simulink library "lineAngleSensorObserver"  (R2022a)
settings: Solver=VariableStepAuto  StartTime=0.0  StopTime=10.0  RelTol=1e-3
undefined symbols (not defined in the file): accelBias, bridlePosVec, env, eulerBias, fluidDensity, gravity, initPosKite, initVelKite, las, NNodeTether, NNodeTether_cl, ObserverGains, obsLASphidotInit, obsLASphiInit, obsLASthetadotInit, obsLASthetaInit, ObsLinkFlowVecsConstant, Obsthr, rampSlope
libraries: lineAngleSensor x4, vrlib x3, sharedtransform x3, sharedutil x3, dspsigops x2, nodeDragForce_ul x1, nodeNetBuoyForce_ul x1, nodePosToLinkPos_ul x1, nodeSpringDamperForce_ul x1, thrNodeMass_ul x1, simulink x1, firstOrdTrnsThm_ul x1
settings Model: Creator=andre  LastModifiedBy=lhill8
settings SolverCC: AlgebraicLoopSolver=TrustRegion
settings DebuggingCC: UnconnectedInputMsg=warning  UnconnectedOutputMsg=warning  UnconnectedLineMsg=warning  SFMachineParentedDataDiag=warning

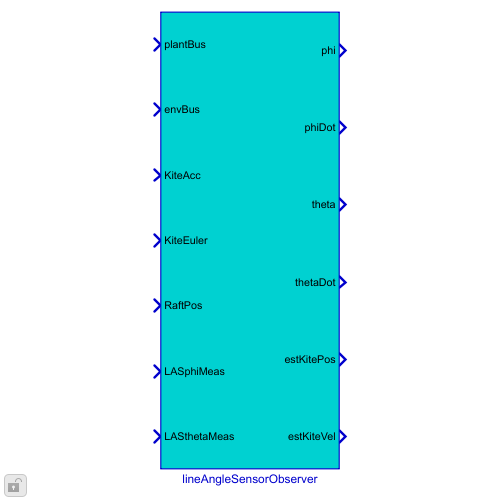
[thumbnail: Simulink's stored preview of the top-level diagram]
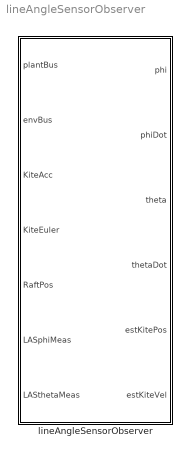
== system lineAngleSensorObserver ==
  lineAngleSensorObserver : Subsystem  mask{las=las, env=env}
      mask prompts: las "LAS Object"; env "Environment"

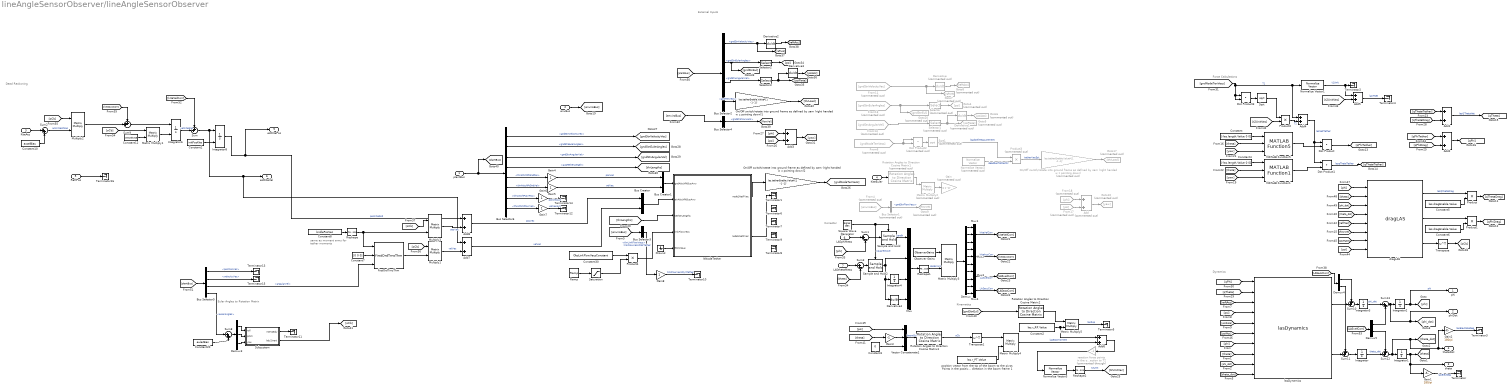
== system lineAngleSensorObserver/lineAngleSensorObserver ==
  note: Euler Angles to Rotation Matrix
  note: Dead Reckoning
  note: Corrector
  note: Kinematics
  note: Force Calculations
  note: Dynamics
  note: External Inputs
  note: same as moment arms
      | for tether moments
  plantBus : Inport
  envBus : Inport  Port=2
  KiteAcc : Inport  Port=3
  KiteEuler : Inport  Port=4
  RaftPos : Inport  Port=5
  LASphiMeas : Inport  Port=6
  LASthetaMeas : Inport  Port=7
  Add : Sum  Commented=on
  Add{1..8} (8 alike) : Sum
  Bus Creator : BusCreator  Inputs=2  OutDataTypeStr=Bus: thrAttachPtKinematicsBus  NonVirtualBus=on
  Bus Creator1 : BusCreator  Inputs=2  OutDataTypeStr=Bus: thrAttachPtKinematicsBus  NonVirtualBus=on
  Bus Selector1 : BusSelector  Commented=on  OutputSignals=gndStnFlowVecs
  Bus Selector2 : BusSelector  OutputSignals=gndStnVelocityVec,gndStnEulerAngles,gndStnAngularVel,gndTenVecs
  Bus Selector3 : BusSelector  OutputSignals=thrLinkFlowVecs
  Bus Selector4 : BusSelector  OutputSignals=gndStnFlowVecs
  Bus Selector5 : BusSelector  OutputSignals=positionVec,velocityVec,angularVel,eulerAngles
  Bus Selector6 : BusSelector  OutputSignals=gndStnVelocityVec,gndStnEulerAngles,gndStnAngularVel,avgTetherLength,thrAttchPtGndPos,thrAttchPtGndVel,thrAttchPtAirPos,thrAttchPtAirVel
  Constant : Constant  Value=[-las.length.Value 0 0]
  Constant1 : Constant  Value=initPosKite
  Constant10 : Constant  Value=accelBias
  Constant12 : Constant  Value=initVelKite
  Constant2 : Constant  Value=las.r_RP.Value
  Constant20 : Constant  Value=eulerBias
  Constant3 : Constant  Value=0
  Constant30 : Constant  Value=ObsLinkFlowVecsConstant
  Constant4 : Constant  Value=[-las.length.Value 0 0]
  Constant5 : Constant  Value=las.dragEnable.Value
  Constant6 : Constant  Value=las.dragEnable.Value
  Constant7 : Constant  Value=[0 0 0]
  Constant8 : Constant  Value=bridlePosVec
  Demux : Demux  Outputs=10
  Demux3 : Demux  Outputs=3
  Demux4 : Demux  Outputs=2
  Demux5 : Demux  Outputs=2
  Derivative : Derivative  Commented=on
  Derivative1 : Derivative  Commented=on
  Derivative2 : Derivative
  Derivative3 : Derivative
  Derivative4 : Derivative
  Dot Product : DotProduct  OutDataTypeStr=Inherit: Inherit via internal rule
  Dot Product1 : DotProduct  OutDataTypeStr=Inherit: Inherit via internal rule
  Dot Product2 : DotProduct  Commented=on  OutDataTypeStr=Inherit: Inherit via internal rule
  Dot Product3 : DotProduct  OutDataTypeStr=Inherit: Inherit via internal rule
  From11 : From  Commented=on  GotoTag=gndStnVelocityVec
  From13 : From  Commented=on  GotoTag=gndStnEulerAngles
  From14 : From  Commented=on  GotoTag=gndStnAngularVel
  From17 : From  Commented=on  GotoTag=psi
  From18 : From  Commented=on  GotoTag=phi
  From4 : From  Commented=on  GotoTag=enviroBus
  From6 : From  Commented=on  GotoTag=gndNodeTenVecs
  Gain : Gain  Commented=on  Gain=[1 1 -1]'
  Gain1 : Gain  Gain=180/pi
  Gain2 : Gain  Gain=180/pi
  Gain3 : Gain  Gain=-1
  Gain{4..8} (5 alike) : Gain
  Goto10 : Goto  Commented=on  GotoTag=yaw
  Goto17 : Goto  Commented=on  GotoTag=thrLoad
  Goto20 : Goto  Commented=on  GotoTag=gndStnEul
  Goto4 : Goto  Commented=on  GotoTag=psi
  Goto5 : Goto  Commented=on  GotoTag=psiRate
  Goto6 : Goto  Commented=on  GotoTag=psiAcc
  Goto7 : Goto  Commented=on  GotoTag=raftVel
  Goto8 : Goto  Commented=on  GotoTag=raftAcc
  Goto9 : Goto  Commented=on  GotoTag=flowVel
  Ground : Ground
  Integrator : Integrator  InitialCondition=obsLASthetadotInit
  Integrator1 : Integrator  InitialCondition=obsLASthetaInit
  Integrator2 : Integrator  InitialCondition=obsLASphiInit
  Integrator3 : Integrator  InitialCondition=obsLASphidotInit
  Integrator4 : Integrator
  Integrator6 : Integrator  InitialConditionSource=external
  Integrator8 : Integrator  InitialConditionSource=external
  MATLAB Function1 : lineAngleSensor/lineAngleSensor/MATLAB Function1  SystemSampleTime=-1  VariantActivationTime=update diagram  Latency=0  AutoFrameSizeCalculation=off
  MATLAB Function5 : lineAngleSensor/lineAngleSensor/MATLAB Function5  SystemSampleTime=-1  VariantActivationTime=update diagram  Latency=0  AutoFrameSizeCalculation=off
  Matrix Multiply{1,3..5} (4 alike) : Product  Multiplication=Matrix(*)
  Matrix Multiply2 : Product  Commented=on  Multiplication=Matrix(*)
  Multiply1 : Product  Multiplication=Matrix(*)
  Multiply2 : Product  Multiplication=Matrix(*)
  Multiply3 : Product  Multiplication=Matrix(*)
  Mux : Mux
  Mux1 : Mux  Inputs=3
  Mux2 : Mux  Inputs=3
  Mux3 : Mux  Inputs=2
  Mux4 : Mux  Inputs=2
  NNodeTether : Subsystem  AncestorBlock=NNodeTether_cl/NNodeTether  VariantControl=NNodeTether  mask{thr=Obsthr.struct('OCT.tether'), flowDensity=fluidDensity, gravity=gravity, numNodes=Obsthr.numNodes.Value}
      mask prompts: thr "Tether Structure"; flowDensity "Fluid Density"; gravity "Gravitational Acceleration"; numNodes "Number of Nodes"
  Normalize Vector1 : vrlib/Utilities/Normalize Vector  maxzero=0
  Normalize Vector2 : vrlib/Utilities/Normalize Vector  Commented=on  maxzero=0
  Normalize Vector3 : vrlib/Utilities/Normalize Vector  maxzero=0
  Observer Gains : Constant  Value=ObserverGains
  On/Off switch/rotate into ground frame as defined by sam (right handed w z pointing down) : Gain  Commented=on  Gain=las.tetherEnable.Value*[1 -1 -1]'
  On/Off switch/rotate into ground frame as defined by sam (right handed w z pointing down)1 : Gain  Gain=las.tetherEnable.Value*[1 -1 -1]'
  On/Off switch/rotate into ground frame as defined by sam (right handed w z pointing down)2 : Gain  Gain=las.tetherEnable.Value*[1 -1 -1]'
  Product{,1..2,4} (4 alike) : Product
  Product3 : Product  Commented=on
  Ramp : simulink/Sources/Ramp  slope=rampSlope  start=0  InitialOutput=0
  Reshape : Reshape  OutputDimensionality=Column vector (2-D)
  Reshape1 : Reshape  OutputDimensionality=Column vector (2-D)
  Reshape2 : Reshape  OutputDimensionality=Column vector (2-D)
  Rotation Angles to Direction Cosine Matrix1 : sharedtransform/Rotation Angles to Direction Cosine Matrix  Commented=on  rotationOrder=ZYX  aMode=aMode
      settings: SourceProductBaseCode=AE,PW,DR,MT,VE
  Rotation Angles to Direction Cosine Matrix2 : sharedtransform/Rotation Angles to Direction Cosine Matrix  rotationOrder=ZYX  aMode=aMode
      settings: SourceProductBaseCode=AE,PW,DR,MT,VE
  Rotation Angles to Direction Cosine Matrix3 : sharedtransform/Rotation Angles to Direction Cosine Matrix  rotationOrder=ZYX  aMode=aMode
      settings: SourceProductBaseCode=AE,PW,DR,MT,VE
  Sample and Hold : dspsigops/Sample and Hold  trig=Rising edge  initCond=0  latchinput=off
  Sample and Hold2 : dspsigops/Sample and Hold  trig=Rising edge  initCond=0  latchinput=off
  Saturation : Saturate  UpperLimit=1  LowerLimit=0
  Selector : Selector  Commented=on  InputPortWidth=3  IndexOptions=Index vector (dialog)  Indices=[3]  OutputSizes=1
  Selector1 : Selector  Commented=on  InputPortWidth=3  IndexOptions=Index vector (dialog)  Indices=[3]  OutputSizes=1
  Selector2 : Selector  InputPortWidth=3  IndexOptions=Index vector (dialog)  Indices=[3]  OutputSizes=1
  Selector3 : Selector  InputPortWidth=3  IndexOptions=Index vector (dialog)  Indices=[3]  OutputSizes=1
  Sqrt : Sqrt
  Sqrt1 : Sqrt  Commented=on
  Square Wave Generator : SignalGenerator  WaveForm=square  Frequency=100
  Subsystem : Subsystem
  Sum{,9..12} (5 alike) : Sum  Inputs=++|
  Sum1 : Sum  Inputs=|+-
  Sum13 : Sum  Inputs=|++
  Sum2 : Sum  Inputs=|++
  Sum3 : Sum  Inputs=|+-
  Sum8 : Sum  Inputs=|++
  Terminator{,1..16} (17 alike) : Terminator
  Transpose : Math  Operator=transpose
  Transpose1 : Math  Operator=transpose
  Vector Concatenate1 : Concatenate  NumInputs=3
  dragLAS : lineAngleSensor/lineAngleSensor/dragLAS  rho=env.water.density.Value  C_D=las.CD.Value  L=las.length.Value  numDx=10  w=las.diameter.Value
  firstOrdTrnsThm : firstOrdTrnsThm_ul/firstOrdTrnsThm  SystemSampleTime=-1  VariantActivationTime=update diagram  Latency=0  AutoFrameSizeCalculation=off
  lasDynamics : lineAngleSensor/lineAngleSensor/lasDynamics  g=env.gravAccel.Value  mass_LAS=las.mass.Value  Fb_LAS=las.volume.Value*env.water.density.Value*env.gravAccel.Value  IxxLAS=las.Ixx.Value  IyyLAS=las.Iyy.Value  IzzLAS=las.Izz.Value  L_CB=las.L_CB.Value  L_CM=las.L_CM.Value
  position vector from the tip of the boom to the pivot. Points in the positive i direction in the boom frame 1 : Constant  Value=las.r_PT.Value
  reaction force points in the opposite direction to T2 : Gain  Commented=through  Gain=-1
  phi : Outport
  phiDot : Outport  Port=2
  theta : Outport  Port=3
  thetaDot : Outport  Port=4
  estKitePos : Outport  Port=5
  estKiteVel : Outport  Port=6
  wires:
  On/Off switch/rotate into ground frame as defined by sam (right handed w z pointing down)/1 -> Goto17/1
  Bus Selector1/1 -> Goto9/1  "<gndStnFlowVecs>"
  Derivative1/1 -> Goto6/1
  Selector1/1 -> Goto5/1, Derivative1/1
  From14/1 -> Selector1/1
  Selector/1 -> Goto4/1
  From13/1 -> Goto20/1, Selector/1
  From11/1 -> Goto7/1, Derivative/1
  Derivative/1 -> Goto8/1
  Add/1 -> Goto10/1
  From18/1 -> Add/1
  From17/1 -> Add/2
  plantBus/1 -> Bus Selector6/1, [plantBus]
  From6/1 -> Dot Product2/2, Dot Product2/1
  Dot Product2/1 -> Sqrt1/1
  Sqrt1/1 -> Product3/1  "loadCellMeasurement"
  Normalize Vector2/1 -> Product3/2  "deadRecTetherDir"
  KiteEuler/1 -> Rotation Angles to Direction Cosine Matrix1/1
  Rotation Angles to Direction Cosine Matrix1/1 -> Matrix Multiply2/1
  Matrix Multiply2/1 -> Gain/1
  Observer Gains/1 -> Matrix Multiply3/1
  [phi] -> Sum1/2
  LASphiMeas/1 -> Sum1/1
  LASthetaMeas/1 -> Sum3/1
  [theta] -> Sum3/2
  Sum3/1 -> Sample and Hold2/1
  Sample and Hold/1 -> Mux/1  "sandh"
  Mux/1 -> Reshape1/1
  Reshape1/1 -> Matrix Multiply3/2  "obsErrors"
  Matrix Multiply3/1 -> Demux/1
  Demux/1 -> Mux1/1
  Demux/2 -> Mux1/2
  Demux/3 -> Mux1/3
  Demux/7 -> Mux3/1
  Demux/8 -> Mux3/2
  Demux/9 -> Mux4/1
  Demux/10 -> Mux4/2
  Mux1/1 -> [kiteVelCorr]  "kiteVelCorr"
  Demux/4 -> Mux2/1
  Demux/5 -> Mux2/2
  Demux/6 -> Mux2/3
  Mux2/1 -> [kiteAccCorr]  "kiteAccCorr"
  Mux4/1 -> [LASaccCorr]  "LASaccCorr"
  Mux3/1 -> [LASvelCorr]  "LASvelCorr"
  Rotation Angles to Direction Cosine Matrix3/1 -> Transpose1/1  "oCb"
  [psi] -> Vector Concatenate1/1
  [gndStnEul] -> Rotation Angles to Direction Cosine Matrix2/1
  Rotation Angles to Direction Cosine Matrix2/1 -> Matrix Multiply5/1
  reaction force points in the opposite direction to T2/1 -> Normalize Vector3/1
  Reshape2/1 -> [t2UnitVec]  "t2Unit"
  Constant2/1 -> Add6/1, Matrix Multiply5/2
  Gain3/1 -> Vector Concatenate1/2
  Vector Concatenate1/1 -> Rotation Angles to Direction Cosine Matrix3/1  "boomEul"
  Constant3/1 -> Vector Concatenate1/3
  position vector from the tip of the boom to the pivot. Points in the positive i direction in the boom frame 1/1 -> Matrix Multiply4/2
  Matrix Multiply4/1 -> Add6/2  "lasBoomOrient"
  Add6/1 -> reaction force points in the opposite direction to T2/1
  Transpose1/1 -> Matrix Multiply4/1
  Matrix Multiply5/1 -> Terminator5/1  "lasRop"
  Normalize Vector3/1 -> Reshape2/1
  [theta] -> Gain3/1
  MATLAB Function5/1 -> Dot Product/2
  Constant/1 -> MATLAB Function5/1
  [theta] -> lasDynamics/8
  [phi] -> dragLAS/1
  [raftAcc] -> lasDynamics/3
  [psi] -> lasDynamics/4
  [psiRate] -> lasDynamics/5
  [theta] -> dragLAS/2
  [phi] -> lasDynamics/7
  [psi] -> dragLAS/8
  lasDynamics/2 -> Sum11/2
  [phi_dot] -> lasDynamics/9
  Integrator1/1 -> Gain1/1, theta/1, [theta]
  Gain2/1 -> Terminator3/1  "lasElevRateDeg"
  [yaw] -> MATLAB Function5/3
  Add1/1 -> [qTheta]  "lasQThetaNet"
  Constant4/1 -> MATLAB Function1/1
  [qPhiDrag] -> Add2/2
  [flowVel] -> dragLAS/6
  Gain1/1 -> Terminator/1  "lasElevDeg"
  [gndNodeTenVecs] -> Dot Product3/2, Dot Product3/1, Normalize Vector1/1, Add4/1  "T1"
  [theta] -> MATLAB Function5/2
  Product/1 -> [qThetaDrag]
  dragLAS/3 -> Transpose/1
  Constant5/1 -> Product/2
  lasDynamics/1 -> Sum10/2
  Product1/1 -> [qPhiDrag]
  Dot Product/1 -> [qPhiTether]
  [raftVel] -> dragLAS/5
  dragLAS/1 -> Product/1  "lasQthetaDrag"
  [t2UnitVec] -> Product2/2
  Add5/1 -> Terminator4/1  "lasTNet"
  Dot Product1/1 -> [qThetaTether]  "lasqThetaTether"
  [t2UnitVec] -> Add5/2
  Integrator2/1 -> phi/1, [phi]  "phi"
  [qThetaTether] -> Add1/1
  [phi_dot] -> dragLAS/3
  [theta_dot] -> lasDynamics/10
  Product2/1 -> Add4/2  "T2"
  [yaw] -> MATLAB Function1/3
  Dot Product3/1 -> Sqrt/1
  [theta_dot] -> dragLAS/4
  [psiRate] -> dragLAS/7
  [qPhi] -> lasDynamics/1
  MATLAB Function1/1 -> Dot Product1/2
  [theta] -> MATLAB Function1/2
  Add2/1 -> [qPhi]
  [psiAcc] -> lasDynamics/6
  Constant6/1 -> Product1/2
  Sqrt/1 -> Product2/1
  Add4/1 -> Dot Product1/1, Dot Product/1  "lasNetTether"
  dragLAS/2 -> Product1/1
  Sum12/1 -> Gain2/1, thetaDot/1, [theta_dot], Integrator1/1
  [qThetaDrag] -> Add1/2
  Transpose/1 -> [oCb]
  Normalize Vector1/1 -> Add5/1, Terminator2/1  "t1Unit"
  [qPhiTether] -> Add2/1
  Sum13/1 -> Integrator2/1, phiDot/1, [phi_dot]
  [qTheta] -> lasDynamics/2
  Product3/1 -> On/Off switch/rotate into ground frame as defined by sam (right handed w z pointing down)/1  "tetherVecEst"
  [enviroBus] -> Bus Selector3/1
  envBus/1 -> [enviroBus]
  From4/1 -> Bus Selector1/1
  Ground/1 -> NNodeTether/5(fltCtrlBus)
  NNodeTether/1(node1NetFVec) -> On/Off switch/rotate into ground frame as defined by sam (right handed w z pointing down)2/1
  NNodeTether/2(nodeNNetFVec) -> Terminator1/1
  ? -> Terminator7/1
  ? -> Terminator8/1
  ? -> Terminator9/1
  Bus Selector6/1 -> [gndStnVelocityVec]  "<gndStnVelocityVec>"
  Bus Selector6/2 -> [gndStnEulerAngles]  "<gndStnEulerAngles>"
  Bus Selector6/3 -> [gndStnAngularVel]  "<gndStnAngularVel>"
  Bus Selector6/4 -> [thrLengths]  "<avgTetherLength>"
  [thrLengths] -> NNodeTether/3(tetherLengths)
  Add8/1 -> Bus Creator/1  "posVec"
  Add7/1 -> Bus Creator/2  "velVec"
  Bus Selector4/1 -> [flowVel]  "<gndStnFlowVecs>"
  [psi] -> Add3/2
  Bus Selector2/2 -> [gndStnEul], Selector2/1  "<gndStnEulerAngles>"
  Add3/1 -> [yaw]
  [plantBus] -> Bus Selector2/1
  On/Off switch/rotate into ground frame as defined by sam (right handed w z pointing down)1/1 -> [thrLoad]
  Bus Selector2/1 -> Derivative2/1, [raftVel]  "<gndStnVelocityVec>"
  [phi] -> Add3/1
  Derivative3/1 -> [psiAcc]
  Selector3/1 -> Derivative3/1, [psiRate]
  [enviroBus] -> Bus Selector4/1
  Derivative2/1 -> [raftAcc]
  Bus Selector2/3 -> Selector3/1  "<gndStnAngularVel>"
  Selector2/1 -> [psi]
  Bus Selector2/4 -> On/Off switch/rotate into ground frame as defined by sam (right handed w z pointing down)1/1  "<gndTenVecs>"
  ? -> Terminator6/1  "nodePosVecs"
  RaftPos/1 -> Terminator16/1
  Gain4/1 -> Bus Creator1/1  "posVec"
  Gain5/1 -> Bus Creator1/2  "velVec"
  Demux3/1 -> Subsystem/1(roll)
  Demux3/3 -> Subsystem/3(yaw)
  Demux3/2 -> Subsystem/2(pitch)
  [plantBus] -> Bus Selector5/1
  Bus Selector5/3 -> firstOrdTrnsThm/3  "<angularVel>"
  Bus Selector5/4 -> Sum8/1  "<eulerAngles>"
  Bus Creator1/1 -> NNodeTether/1(gndAttchPtBusArry)
  Bus Creator/1 -> NNodeTether/2(airAttchPtBusArry)
  Reshape/1 -> firstOrdTrnsThm/1, Multiply3/2
  firstOrdTrnsThm/1 -> Multiply1/2
  Constant8/1 -> Reshape/1
  Constant7/1 -> firstOrdTrnsThm/2
  Multiply3/1 -> Add8/2  "posVec"
  Multiply1/1 -> Add7/2  "velVec"
  Gain6/1 -> Terminator14/1  "posVecAct"
  Gain7/1 -> Terminator12/1  "velVecAct"
  Subsystem/1(inert2Bdy) -> Terminator11/1
  Bus Selector6/7 -> Gain6/1  "<thrAttchPtAirPos>"
  Bus Selector6/8 -> Gain7/1  "<thrAttchPtAirVel>"
  Bus Selector6/5 -> Gain4/1  "<thrAttchPtGndPos>"
  Bus Selector6/6 -> Gain5/1  "<thrAttchPtGndVel>"
  Integrator8/1 -> Add8/1, estKitePos/1  "posKiteGnd"
  Sum2/1 -> Multiply2/2  "accKiteWbias"
  Bus Selector5/1 -> Terminator13/1  "<positionVec>"
  Bus Selector5/2 -> Terminator15/1  "<velocityVec>"
  Sum1/1 -> Sample and Hold/1
  Sample and Hold2/1 -> Derivative4/1, Integrator4/1, Mux/2
  Square Wave Generator/1 -> Sample and Hold/Trigger, Sample and Hold2/Trigger  "squareWave"
  On/Off switch/rotate into ground frame as defined by sam (right handed w z pointing down)2/1 -> [gndNodeTenVecs]
  Integrator4/1 -> Mux/3
  Matrix Multiply1/1 -> Integrator6/2
  Constant12/1 -> Matrix Multiply1/2
  Subsystem/2(bdy2Inert) -> [oCb]
  Constant1/1 -> Integrator8/2
  Sum/1 -> Add7/1, estKiteVel/1, Integrator8/1
  [kiteVelCorr] -> Sum/1
  Integrator6/1 -> Sum/2  "velKiteGnd"
  KiteAcc/1 -> Sum2/1
  Constant10/1 -> Sum2/2
  Derivative4/1 -> Mux/4
  Sum8/1 -> Demux3/1
  Constant20/1 -> Sum8/2
  Sum9/1 -> Integrator6/1
  [kiteAccCorr] -> Sum9/1
  [LASaccCorr] -> Demux4/1
  Sum10/1 -> Integrator3/1
  Demux4/1 -> Sum10/1
  Sum11/1 -> Integrator/1
  Demux4/2 -> Sum11/1
  [LASvelCorr] -> Demux5/1
  Integrator/1 -> Sum12/2  "theta_dot"
  Demux5/2 -> Sum12/1
  Integrator3/1 -> Sum13/1  "phi_dot"
  Demux5/1 -> Sum13/2
  Constant30/1 -> Product4/1
  Product4/1 -> NNodeTether/4(linkFlowVecs)  "linkFlowVecsObsTether"
  Ramp/1 -> Saturation/1
  Saturation/1 -> Product4/2
  Bus Selector3/1 -> Gain8/1  "<thrLinkFlowVecs>"
  Gain8/1 -> Terminator10/1  "linkFlowVecsDynTether"
  [oCb] -> Multiply1/1
  [oCb] -> Multiply3/1
  [oCb] -> Matrix Multiply1/1
  [oCb] -> Multiply2/1
  Multiply2/1 -> Sum9/2

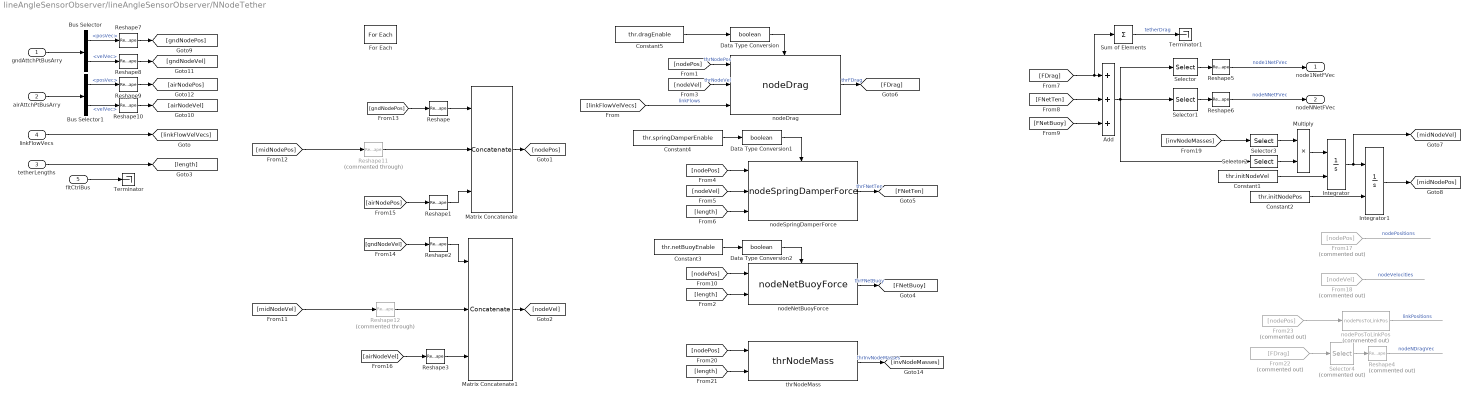
== system lineAngleSensorObserver/lineAngleSensorObserver/NNodeTether ==
  gndAttchPtBusArry : Inport  OutDataTypeStr=Bus: thrAttachPtKinematicsBus  Partition=on  PartitionDimension=1  PartitionWidth=1  PartitionOffset=0
  airAttchPtBusArry : Inport  Port=2  OutDataTypeStr=Bus: thrAttachPtKinematicsBus  Partition=on  PartitionDimension=1  PartitionWidth=1  PartitionOffset=0
  tetherLengths : Inport  Port=3  Partition=on  PartitionDimension=1  PartitionWidth=1  PartitionOffset=0
  linkFlowVecs : Inport  Port=4  Partition=on  PartitionDimension=3  PartitionWidth=1  PartitionOffset=0
  fltCtrlBus : Inport  Port=5
  Add : Sum  Inputs=3
  Bus Selector : BusSelector  OutputSignals=posVec,velVec
  Bus Selector1 : BusSelector  OutputSignals=posVec,velVec
  Constant1 : Constant  Value=thr.initNodeVel
  Constant2 : Constant  Value=thr.initNodePos
  Constant3 : Constant  Value=thr.netBuoyEnable
  Constant4 : Constant  Value=thr.springDamperEnable
  Constant5 : Constant  Value=thr.dragEnable
  Data Type Conversion : DataTypeConversion  OutDataTypeStr=boolean  SaturateOnIntegerOverflow=off  RndMeth=Floor
  Data Type Conversion1 : DataTypeConversion  OutDataTypeStr=boolean  SaturateOnIntegerOverflow=off  RndMeth=Floor
  Data Type Conversion2 : DataTypeConversion  OutDataTypeStr=boolean  SaturateOnIntegerOverflow=off  RndMeth=Floor
  For Each : ForEach  DisableCoverage=on  IterateSubsysMaskParameter=off,off,off,off  SubsysMaskParameterIterationDimension=1,1,1,1  SubsysMaskParameterIterationStepSize=1,1,1,1
  From17 : From  Commented=on  GotoTag=nodePos
  From18 : From  Commented=on  GotoTag=nodeVel
  From22 : From  Commented=on  GotoTag=FDrag
  From23 : From  Commented=on  GotoTag=nodePos
  Integrator : Integrator  InitialConditionSource=external
  Integrator1 : Integrator  InitialConditionSource=external
  Matrix Concatenate : Concatenate  NumInputs=3  Mode=Multidimensional array  ConcatenateDimension=2
  Matrix Concatenate1 : Concatenate  NumInputs=3  Mode=Multidimensional array  ConcatenateDimension=2
  Multiply : Product
  Reshape{,1..3,5..10} (10 alike) : Reshape  OutputDimensionality=Column vector (2-D)
  Reshape11 : Reshape  Commented=through  OutputDimensionality=Column vector (2-D)
  Reshape12 : Reshape  Commented=through  OutputDimensionality=Column vector (2-D)
  Reshape4 : Reshape  Commented=on  OutputDimensionality=Column vector (2-D)
  Selector : Selector  NumberOfDimensions=2  InputPortWidth=3  IndexOptions=Select all,Index vector (dialog)  Indices=[1 3],1  OutputSizes=1,1
  Selector1 : Selector  NumberOfDimensions=2  InputPortWidth=3  IndexOptions=Select all,Starting index (dialog)  Indices=[1 3],numNodes  OutputSizes=1,1
  Selector2 : Selector  NumberOfDimensions=2  InputPortWidth=3  IndexOptions=Select all,Index vector (dialog)  Indices=[1 3],2:numNodes-1  OutputSizes=1,1
  Selector3 : Selector  NumberOfDimensions=2  InputPortWidth=3  IndexOptions=Select all,Index vector (dialog)  Indices=[1 3],2:numNodes-1  OutputSizes=1,1
  Selector4 : Selector  Commented=on  NumberOfDimensions=2  InputPortWidth=3  IndexOptions=Select all,Starting index (dialog)  Indices=[1 3],numNodes  OutputSizes=1,1
  Sum of Elements : Sum  Inputs=+  CollapseMode=Specified dimension  CollapseDim=2
  Terminator : Terminator
  Terminator1 : Terminator
  nodeDrag : nodeDragForce_ul/nodeDrag  flowDensity=flowDensity  thrDiam=thr.diameter  dragCoeff=thr.dragCoeff
  nodeNetBuoyForce : nodeNetBuoyForce_ul/nodeNetBuoyForce  fluidDensity=flowDensity  tetherDensity=thr.density  diameter=thr.diameter  gravity=gravity
  nodePosToLinkPos : nodePosToLinkPos_ul/nodePosToLinkPos  Commented=on  SystemSampleTime=-1  VariantActivationTime=update diagram  Latency=0  AutoFrameSizeCalculation=off
  nodeSpringDamperForce : nodeSpringDamperForce_ul/nodeSpringDamperForce  mass=thr.vehicleMass  zeta=thr.dampingRatio  diameter=thr.diameter  youngsMod=thr.youngsMod
  thrNodeMass : thrNodeMass_ul/thrNodeMass  tetherDensity=thr.density  diameter=thr.diameter
  node1NetFVec : Outport  ConcatenationDimension=3  VectorParamsAs1DForOutWhenUnconnected=off
  nodeNNetFVec : Outport  Port=2  ConcatenationDimension=3  VectorParamsAs1DForOutWhenUnconnected=off
  wires:
  linkFlowVecs/1 -> [linkFlowVelVecs]
  [linkFlowVelVecs] -> nodeDrag/3  "linkFlows"
  Constant5/1 -> Data Type Conversion/1
  Sum of Elements/1 -> Terminator1/1  "tetherDrag"
  fltCtrlBus/1 -> Terminator/1
  Reshape4/1 -> ?  "nodeNDragVec"
  From22/1 -> Selector4/1
  Selector4/1 -> Reshape4/1
  nodePosToLinkPos/1 -> ?  "linkPositions"
  From18/1 -> ?  "nodeVelocities"
  From17/1 -> ?  "nodePositions"
  Reshape6/1 -> nodeNNetFVec/1  "nodeNNetFVec"
  Reshape5/1 -> node1NetFVec/1  "node1NetFVec"
  From23/1 -> nodePosToLinkPos/1
  thrNodeMass/1 -> [invNodeMasses]  "thrInvNodeMasses"
  [length] -> thrNodeMass/2
  [nodePos] -> thrNodeMass/1
  Matrix Concatenate1/1 -> [nodeVel]
  [invNodeMasses] -> Selector3/1
  Selector3/1 -> Multiply/1
  Constant2/1 -> Integrator1/2
  Constant1/1 -> Integrator/2
  Data Type Conversion/1 -> nodeDrag/Enable
  Data Type Conversion1/1 -> nodeSpringDamperForce/Enable
  Constant4/1 -> Data Type Conversion1/1
  Constant3/1 -> Data Type Conversion2/1
  Data Type Conversion2/1 -> nodeNetBuoyForce/Enable
  Multiply/1 -> Integrator/1
  Reshape8/1 -> [gndNodeVel]
  Bus Selector/1 -> Reshape7/1  "<posVec>"
  Bus Selector1/2 -> Reshape10/1  "<velVec>"
  Reshape7/1 -> [gndNodePos]
  Reshape9/1 -> [airNodePos]
  Bus Selector1/1 -> Reshape9/1  "<posVec>"
  tetherLengths/1 -> [length]
  gndAttchPtBusArry/1 -> Bus Selector/1
  Bus Selector/2 -> Reshape8/1  "<velVec>"
  airAttchPtBusArry/1 -> Bus Selector1/1
  Reshape10/1 -> [airNodeVel]
  Matrix Concatenate/1 -> [nodePos]
  [midNodePos] -> Reshape11/1
  Integrator1/1 -> [midNodePos]
  Integrator/1 -> [midNodeVel], Integrator1/1
  Selector2/1 -> Multiply/2
  [gndNodePos] -> Reshape/1
  [gndNodeVel] -> Reshape2/1
  [airNodePos] -> Reshape1/1
  [airNodeVel] -> Reshape3/1
  Reshape/1 -> Matrix Concatenate/1
  Reshape1/1 -> Matrix Concatenate/3
  Reshape3/1 -> Matrix Concatenate1/3
  Reshape2/1 -> Matrix Concatenate1/1
  [nodePos] -> nodeDrag/1  "thrNodePos"
  [length] -> nodeNetBuoyForce/2
  [nodeVel] -> nodeDrag/2  "thrNodeVel"
  [nodeVel] -> nodeSpringDamperForce/2
  [nodePos] -> nodeSpringDamperForce/1
  [length] -> nodeSpringDamperForce/3
  nodeNetBuoyForce/1 -> [FNetBuoy]  "thrFNetBuoy"
  nodeSpringDamperForce/1 -> [FNetTen]  "thrFNetTen"
  nodeDrag/1 -> [FDrag]  "thrFDrag"
  [FNetTen] -> Add/2
  [FDrag] -> Add/1, Sum of Elements/1
  [FNetBuoy] -> Add/3
  Selector/1 -> Reshape5/1
  Add/1 -> Selector/1, Selector2/1, Selector1/1
  Selector1/1 -> Reshape6/1
  [nodePos] -> nodeNetBuoyForce/1
  Reshape11/1 -> Matrix Concatenate/2
  Reshape12/1 -> Matrix Concatenate1/2
  [midNodeVel] -> Reshape12/1

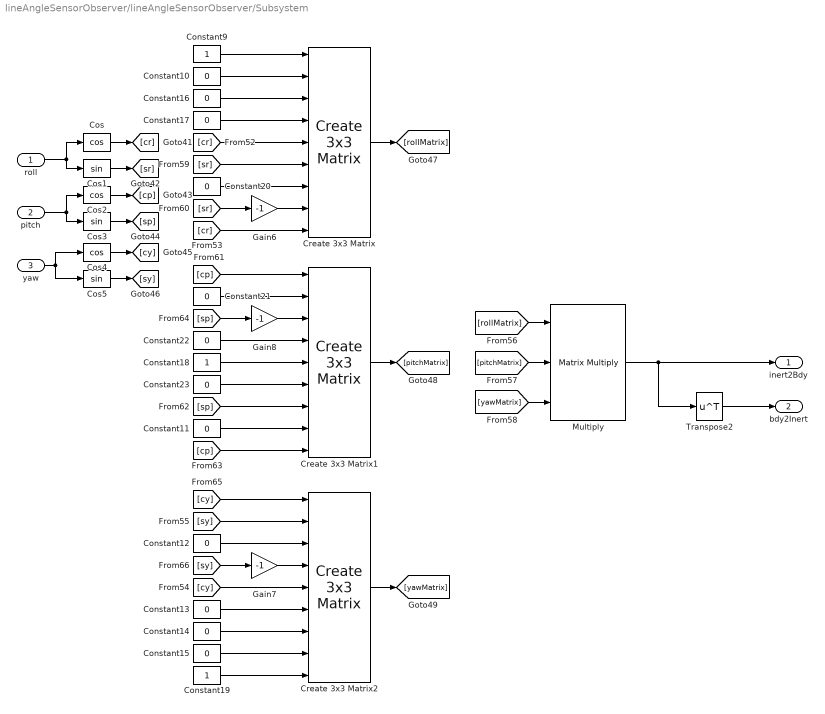
== system lineAngleSensorObserver/lineAngleSensorObserver/Subsystem ==
  roll : Inport
  pitch : Inport  Port=2
  yaw : Inport  Port=3
  Constant{10..17,20..23} (12 alike) : Constant  Value=0
  Constant18 : Constant
  Constant19 : Constant
  Constant9 : Constant
  Cos : Trigonometry  Operator=cos
  Cos1 : Trigonometry
  Cos2 : Trigonometry  Operator=cos
  Cos3 : Trigonometry
  Cos4 : Trigonometry  Operator=cos
  Cos5 : Trigonometry
  Create 3x3 Matrix : sharedutil/Create 3x3 Matrix  aMode=aMode
      settings: SourceProductBaseCode=AE,PW,DR,MT,VE
  Create 3x3 Matrix1 : sharedutil/Create 3x3 Matrix  aMode=aMode
      settings: SourceProductBaseCode=AE,PW,DR,MT,VE
  Create 3x3 Matrix2 : sharedutil/Create 3x3 Matrix  aMode=aMode
      settings: SourceProductBaseCode=AE,PW,DR,MT,VE
  Gain6 : Gain  Gain=-1
  Gain7 : Gain  Gain=-1
  Gain8 : Gain  Gain=-1
  Multiply : Product  Inputs=3  Multiplication=Matrix(*)
  Transpose2 : Math  Operator=transpose  SignedPower=on
  inert2Bdy : Outport  VectorParamsAs1DForOutWhenUnconnected=off
  bdy2Inert : Outport  Port=2  VectorParamsAs1DForOutWhenUnconnected=off
  wires:
  Cos5/1 -> [sy]
  Transpose2/1 -> bdy2Inert/1
  Constant12/1 -> Create 3x3 Matrix2/3
  [cy] -> Create 3x3 Matrix2/5
  [rollMatrix] -> Multiply/1
  Cos2/1 -> [cp]
  [sr] -> Create 3x3 Matrix/6
  [sy] -> Gain7/1
  Create 3x3 Matrix2/1 -> [yawMatrix]
  [cr] -> Create 3x3 Matrix/9
  yaw/1 -> Cos5/1, Cos4/1
  [sp] -> Gain8/1
  Cos4/1 -> [cy]
  Constant17/1 -> Create 3x3 Matrix/4
  Create 3x3 Matrix/1 -> [rollMatrix]
  [cy] -> Create 3x3 Matrix2/1
  [sr] -> Gain6/1
  Constant10/1 -> Create 3x3 Matrix/2
  Constant22/1 -> Create 3x3 Matrix1/4
  Constant16/1 -> Create 3x3 Matrix/3
  Gain7/1 -> Create 3x3 Matrix2/4
  Constant13/1 -> Create 3x3 Matrix2/6
  Constant21/1 -> Create 3x3 Matrix1/2
  Constant15/1 -> Create 3x3 Matrix2/8
  [cp] -> Create 3x3 Matrix1/9
  roll/1 -> Cos1/1, Cos/1
  Multiply/1 -> inert2Bdy/1, Transpose2/1
  Gain6/1 -> Create 3x3 Matrix/8
  Constant11/1 -> Create 3x3 Matrix1/8
  Constant14/1 -> Create 3x3 Matrix2/7
  Constant19/1 -> Create 3x3 Matrix2/9
  Create 3x3 Matrix1/1 -> [pitchMatrix]
  [sp] -> Create 3x3 Matrix1/7
  Constant18/1 -> Create 3x3 Matrix1/5
  Gain8/1 -> Create 3x3 Matrix1/3
  Constant20/1 -> Create 3x3 Matrix/7
  Cos1/1 -> [sr]
  [sy] -> Create 3x3 Matrix2/2
  [yawMatrix] -> Multiply/3
  pitch/1 -> Cos2/1, Cos3/1
  [pitchMatrix] -> Multiply/2
  Cos3/1 -> [sp]
  Constant9/1 -> Create 3x3 Matrix/1
  Constant23/1 -> Create 3x3 Matrix1/6
  [cr] -> Create 3x3 Matrix/5
  Cos/1 -> [cr]
  [cp] -> Create 3x3 Matrix1/1
